simulink model "simulink_Motor_Velocidad"  (R2019a)
settings: Solver=VariableStepAuto  StartTime=0.0  StopTime=10.0  RelTol=1e-3
values from neighbouring files (symbols this model uses):
  Control_z = filt(num,den,Ts)    [AUTO.m]
undefined symbols (not defined in the file or in its folder): F_z
settings Model: Creator=Nahuel  LastModifiedBy=Nahuel

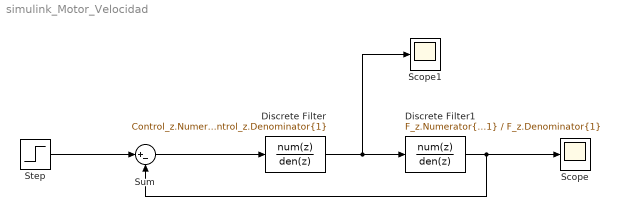
== system simulink_Motor_Velocidad ==
  Discrete Filter : DiscreteFilter  Numerator=Control_z.Numerator{1}  Denominator=Control_z.Denominator{1}
  Discrete Filter1 : DiscreteFilter  Numerator=F_z.Numerator{1}  Denominator=F_z.Denominator{1}
  Scope : Scope
  Scope1 : Scope
  Step : Step  After=261  SampleTime=0
  Sum : Sum  Inputs=|+-
  wires:
  Step/1 -> Sum/1
  Sum/1 -> Discrete Filter/1
  Discrete Filter/1 -> Scope1/1, Discrete Filter1/1
  Discrete Filter1/1 -> Scope/1, Sum/2
